simulink model "Mass_Spring_Damper_System"  (R2025b)
settings: Solver=FixedStepAuto  StartTime=0.0  StopTime=tspan  FixedStep=dt  RelTol=1e-3
values from neighbouring files (symbols this model uses):
  b = transpose(1:10)    [TestLoop.m]    (also in init.m = 1)
  dt_data = round((dt_data_target/dt))*dt    [init.m]
  k = transpose(1:10)    [TestLoop.m]    (also in init.m = 1)
  m = transpose(1:10)    [TestLoop.m]    (also in init.m = 1)
  v0 = transpose(1:10)    [TestLoop.m]    (also in init.m = 0)
  x0 = transpose(1:10)    [TestLoop.m]    (also in init.m = 0)
  y = @(x) 1./x.*sin(x)    [Rank_Parameter.m]    (also in Repeater.m = str2double(get_param(blk,block_parameter)); rank_Parameter.m)
settings Model: Creator=ajosh  LastModifiedBy=ajosh

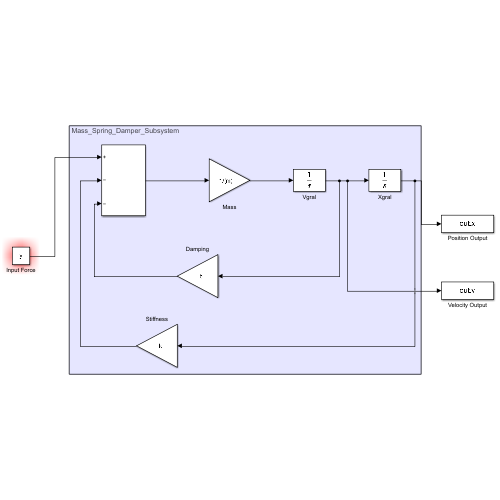
[thumbnail: Simulink's stored preview of the top-level diagram]
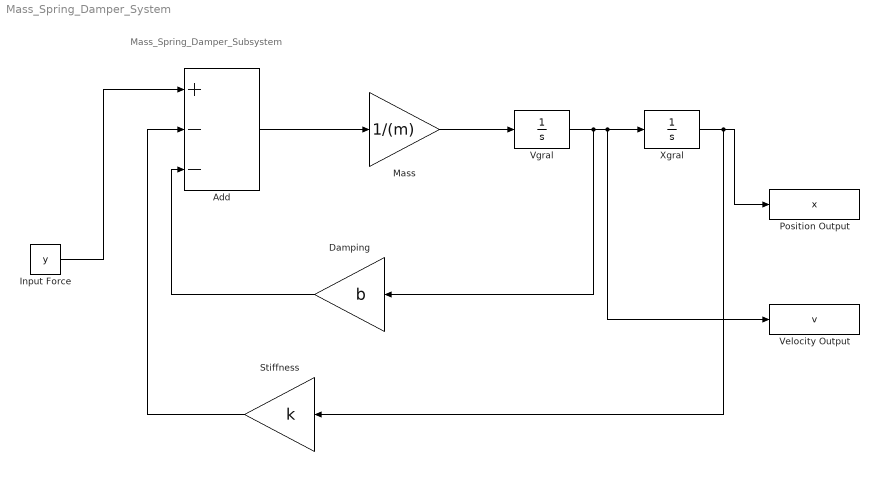
== system Mass_Spring_Damper_System ==
  note: Mass_Spring_Damper_Subsystem
  Add : Sum  Inputs=+--
  Damping : Gain  Gain=b
  Input Force : Constant  Value=y
  Mass : Gain  Gain=1/(m)
  Position Output : ToWorkspace  VariableName=x  SaveFormat=Timeseries  SampleTime=dt_data
  Stiffness : Gain  Gain=k
  Velocity Output : ToWorkspace  VariableName=v  SaveFormat=Timeseries  SampleTime=dt_data
  Vgral : Integrator  InitialCondition=v0
  Xgral : Integrator  InitialCondition=x0
  wires:
  Vgral/1 -> Velocity Output/1, Xgral/1, Damping/1
  Xgral/1 -> Position Output/1, Stiffness/1
  Input Force/1 -> Add/1
  Add/1 -> Mass/1
  Stiffness/1 -> Add/2
  Damping/1 -> Add/3
  Mass/1 -> Vgral/1
